simulink model "ActuatorTest_Example_ToFile"  (R2017b)
settings: Solver=ode4  StartTime=0.0  StopTime=50  FixedStep=0.0025  RelTol=1e-3  AbsTol=1e-6
libraries: DABLib x3
settings Model: Creator=davidlaredorazo  LastModifiedBy=davidlaredorazo
settings DataIOCC: SaveFormat=Array  SignalLoggingSaveFormat=ModelDataLogs
settings OptimizationCC: BlockReduction=off  BooleanDataType=off
settings DebuggingCC: SaveWithParameterizedLinksMsg=none  UnderspecifiedInitializationDetection=Classic  MergeDetectMultiDrivingBlocksExec=none  SignalResolutionControl=TryResolveAllWithWarning  MultiTaskDSMMsg=warning  MultiTaskCondExecSysMsg=none
settings HardwareCC: TargetUnknown=on
settings ModelReferenceCC: PropagateSignalLabelsOutOfModel=off
settings CodeAppCC: StateflowObjectComments=on
settings GRTTargetCC: TargetLangStandard=C89/C90 (ANSI)  CombineOutputUpdateFcns=off  GRTInterface=on

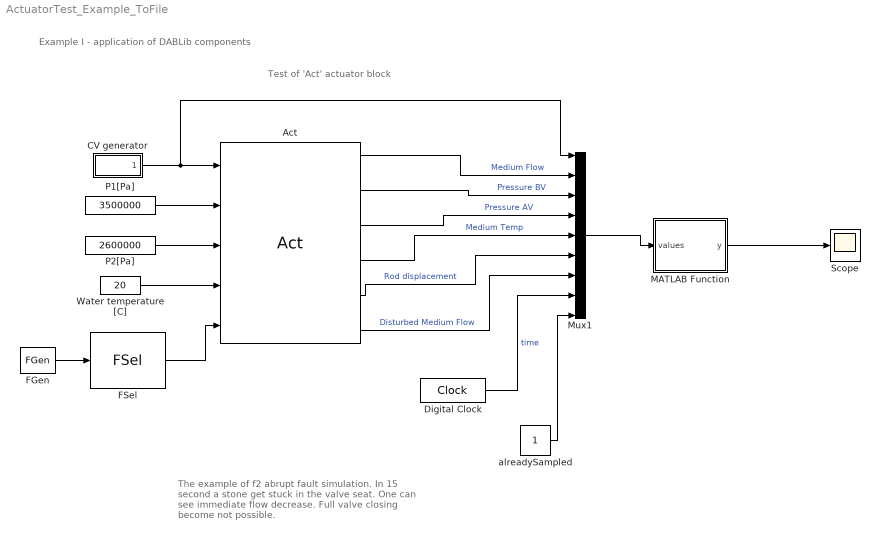
== system ActuatorTest_Example_ToFile ==
  note: Test of 'Act' actuator block
  note: Example I - application of DABLib components
  note: The example of f2 abrupt fault simulation.
      | In 15 second a stone get stuck in the valve seat.
      | One can see immediate flow decrease.
      |  Full valve closing become not possible.
  Act : DABLib/Act  Dist=off
  CV generator : Subsystem
  Digital Clock : DigitalClock
  FGen : DABLib/FGen  From=15  To=inf  MFS=1  FDT=0  FSD=1
  FSel : DABLib/FSel  FSel=f2 - Valve plug or valve seat sedimentation
  MATLAB Function : MATLAB Function  TreatAsAtomicUnit=on
  Mux1 : Mux  Inputs=9
  "P1[Pa] " : Constant  Value=3500000
  "P2[Pa] " : Constant  Value=2600000
  Scope : Scope
  Water temperature [C] : Constant  Value=20
  alreadySampled : Constant  VectorParams1D=off
  wires:
  Mux1/1 -> MATLAB Function/1(values)
  FGen/1 -> FSel/1
  CV generator/1(CV[0-1]) -> Mux1/1, Act/1
  "P1[Pa] "/1 -> Act/2
  "P2[Pa] "/1 -> Act/3
  Water temperature [C]/1 -> Act/4
  Act/2 -> Mux1/3  "Pressure BV"
  Act/3 -> Mux1/4  "Pressure AV"
  Act/4 -> Mux1/5  "Medium Temp"
  Act/6 -> Mux1/7  "Disturbed Medium Flow"
  Act/1 -> Mux1/2  "Medium Flow"
  Act/5 -> Mux1/6  "Rod displacement"
  FSel/1 -> Act/5
  Digital Clock/1 -> Mux1/8  "time"
  alreadySampled/1 -> Mux1/9
  MATLAB Function/1(y) -> Scope/1

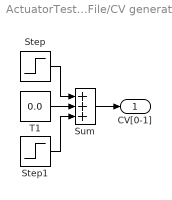
== system ActuatorTest_Example_ToFile/CV generator ==
  Step : Step  Time=0  After=0.5
  Step1 : Step  Time=25  After=0.5
  Sum : Sum  Inputs=+++  SaturateOnIntegerOverflow=on  InputSameDT=on  OutDataTypeStr=Inherit: Same as first input
  T1 : Constant  Value=0.0
  CV[0-1] : Outport  InitialOutput=0
  wires:
  Step/1 -> Sum/1
  T1/1 -> Sum/2
  Step1/1 -> Sum/3
  Sum/1 -> CV[0-1]/1

== matlab function ActuatorTest_Example_ToFile/MATLAB Function ==
  data: values input; y output
function y = saveToDB(values)

coder.extrinsic('set_param');
coder.extrinsic('evalin');
coder.extrinsic('disp');

alreadySampled = values(9);
time = values(8);

%Write samples to the database
if mod(time,5) == 0 && alreadySampled == 0
    set_param('ActuatorTest_Example_ToFile/alreadySampled', 'Value', '1');
    alreadySampled = 1;
    conn = evalin('base', 'dbconn');
    writeToDB(conn, values(1:8));
elseif alreadySampled == 1 && mod(time,5) ~= 0
    set_param('ActuatorTest_Example_ToFile/alreadySampled', 'Value', '0');
    alreadySampled = 0;
end

y = alreadySampled;

end

function writeToDB(dbConn, values)

    coder.extrinsic('evalin');
    coder.extrinsic('sprintf');
    coder.extrinsic('datestr');
    coder.extrinsic('exec');
    coder.extrinsic('fastinsert');

    externalControllerOutput = values(1);
    undisturbedMediumFlow = values(2);
    pressureValveInlet = values(3);
    pressureValveOutlet = values(4);
    mediumTemperature = values(5);
    rodDisplacement = values(6);
    disturbedMediumFlow = values(7);
    elapsedSecond = values(8);
    startDateTime = evalin('base', 'today');
    
    currentDateTime = updateDateTime(startDateTime, elapsedSecond);
    
    %fastinsert(dbConn,'valveReadings', colNames, insertdata)
    
    query = sprintf("INSERT INTO valveReadings(timestamp, externalControllerOutput, undisturbedMediumFlow, "+...
    "pressureValveInlet, pressureValveOutlet, mediumTemperature, rodDisplacement, disturbedMediumFlow) VALUES ('%s', %f, %f, %f," + ...  
    " %f, %f, %f, %f);", datestr(currentDateTime, 'yyyy-mm-dd HH:MM:SS'), externalControllerOutput, undisturbedMediumFlow, pressureValveInlet, ...
    pressureValveOutlet, mediumTemperature, rodDisplacement, disturbedMediumFlow);
    curs = exec(dbConn, query);
    disp(curs);

end

function currentDateTime = updateDateTime(startDateTime, elapsedSeconds)

    coder.extrinsic('datetime');

    hours = 0;
    minutes = 0;
    seconds = 0;

    days = fix(elapsedSeconds/86400);
    reminder = mod(elapsedSeconds,86400);
    
    if reminder ~= 0
        
        hours = fix(reminder/3600);
        reminder = mod(reminder,3600);
        
        if reminder ~= 0
            minutes = fix(reminder/60);
            seconds = mod(reminder,60);
        end
        
    end
    
    currentDateTime = datetime(2017, 10, days, hours, minutes, seconds, 0);

end
